simulink model "RCAMSimulation"  (R2025a)
settings: Solver=VariableStepAuto  StartTime=0.0  StopTime=60  RelTol=1e-3
values from neighbouring files (symbols this model uses):
  dt = 1/50    (= 0.02)    [InitializeConstants.m]    (also in joystickdemo.m)
  h0 = 500    [InitializeConstants.m]
  lat0 = deg2rad(21.3245)    [InitializeConstants.m]
  lon0 = deg2rad(-157.9251)    [InitializeConstants.m]
  u1max = 25*pi/180    (= 0.436332312999)    [InitializeConstants.m]    (also in RCAM_model.m)
  u1min = -25*pi/180    (= -0.436332312999)    [InitializeConstants.m]    (also in RCAM_model.m)
  x0 = [85 ... (first row only)    [InitializeConstants.m]
undefined symbols (not defined in the file or in its folder): RCAM_model
libraries: aerolibfltsims x2, aerolibanimutils x1
settings Model: Creator=pjpra  LastModifiedBy=pjpra

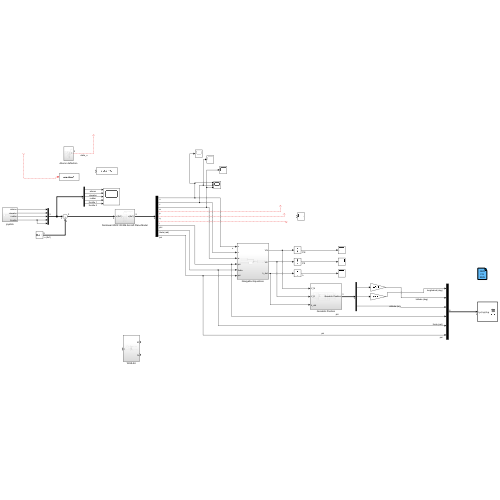
[thumbnail: Simulink's stored preview of the top-level diagram]
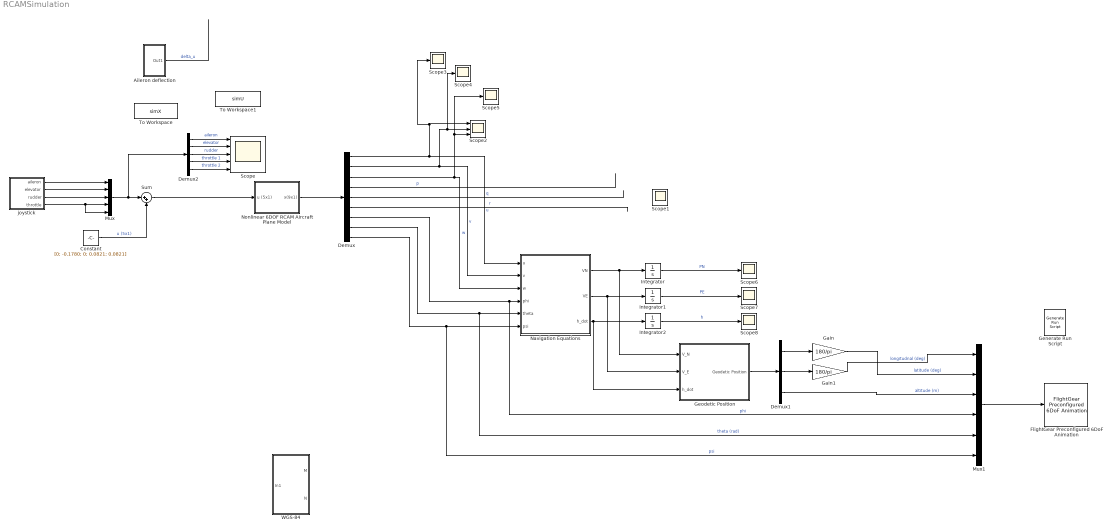
== system RCAMSimulation ==
  Aileron deflection : Subsystem
  Constant : Constant  Value=[0; -0.1780; 0; 0.0821; 0.0821]
  Demux : Demux  Outputs=9
  Demux1 : Demux  Outputs=3
  Demux2 : Demux  Outputs=5
  FlightGear Preconfigured 6DoF Animation : aerolibfltsims/FlightGear Preconfigured 6DoF Animation  xFlightGearVersion=v2019.1  DestinationIpAddress=127.0.0.1  DestinationPort=5502  SampleTime=1/30  packetVersion=24
  Gain : Gain  Gain=180/pi
  Gain1 : Gain  Gain=180/pi
  Generate Run Script : aerolibfltsims/Generate Run Script  Architecture=Win64  dataFlow=Send  GeometryModelName=c172p  AirportId=KSFO  RunwayId=10L  InitialAltitude=7224  InitialHeading=113  OffsetDistance=4.72  OffsetAzimuth=0  InstallScenery=off  DisableShaders=on  OriginAddress=127.0.0.1  DestinationPort=5502  OriginPort=5505  LocalAddress=127.0.0.1  OutputFileName=runfg.bat  FlightGearBaseDirectory=C:\Program Files\FlightGear 2019.1.1
  Geodetic Position : Subsystem
  Integrator : Integrator
  Integrator1 : Integrator
  Integrator2 : Integrator
  Mux : Mux  Inputs=5
  Mux1 : Mux  Inputs=6
  Navigation Equations : Subsystem
  Nonlinear 6DOF RCAM Aircraft Plane Model : Subsystem
  Scope : Scope  NumInputPorts=5
      settings: ActiveDisplayYMinimum=-1  ActiveDisplayYMaximum=1  DataLoggingVariableName=ScopeData3
  Scope{1,3..8} (7 alike) : Scope
      Scope3 settings: ActiveDisplayYMinimum=-115.46318833968678  ActiveDisplayYMaximum=190.41451704390158  DataLoggingVariableName=ScopeData2
      Scope4 settings: ActiveDisplayYMinimum=-115.46318833968678  ActiveDisplayYMaximum=190.41451704390158  DataLoggingVariableName=ScopeData4
      Scope5 settings: ActiveDisplayYMinimum=-115.46318833968678  ActiveDisplayYMaximum=190.41451704390158  DataLoggingVariableName=ScopeData5
      Scope6 settings: ActiveDisplayYMinimum=-336.04878377704415  ActiveDisplayYMaximum=625.66382781010861  DataLoggingVariableName=ScopeData6
      Scope7 settings: ActiveDisplayYMinimum=-115.46318833968678  ActiveDisplayYMaximum=190.41451704390158  DataLoggingVariableName=ScopeData7
      Scope8 settings: ActiveDisplayYMinimum=-228.9226672413669  ActiveDisplayYMaximum=328.44496651210937  DataLoggingVariableName=ScopeData8
  Scope2 : Scope  NumInputPorts=3
      settings: ActiveDisplayYMinimum=-115.46318833968678  ActiveDisplayYMaximum=190.41451704390158
  Sum : Sum  Inputs=|++
  To Workspace : ToWorkspace  VariableName=simX  SaveFormat=Timeseries  SampleTime=-1
  To Workspace1 : ToWorkspace  VariableName=simU  SaveFormat=Timeseries  SampleTime=-1
  WGS-84 : Subsystem
  joystick : Subsystem
  wires:
  Constant/1 -> Sum/2  "u (5x1)"
  ? -> To Workspace/1
  Sum/1 -> Nonlinear 6DOF RCAM Aircraft Plane Model/1(u (5x1))
  Aileron deflection/1(Out1) -> ?  "delta_u"
  Nonlinear 6DOF RCAM Aircraft Plane Model/1(x(9x1)) -> Demux/1
  Demux/9 -> Mux1/6, Navigation Equations/6(psi)  "psi"
  Demux/7 -> Mux1/4, Navigation Equations/4(phi)  "phi"
  Demux/3 -> Scope5/1, Scope2/3, Navigation Equations/3(w)  "w"
  Demux/2 -> Scope4/1, Scope2/2, Navigation Equations/2(v)  "v"
  Demux/1 -> Scope3/1, Scope2/1, Navigation Equations/1(u)  "u"
  Navigation Equations/1(VN) -> Integrator/1, Geodetic Position/1(V_N)
  Navigation Equations/2(VE) -> Integrator1/1, Geodetic Position/2(V_E)
  Navigation Equations/3(h_dot) -> Geodetic Position/3(h_dot), Integrator2/1
  Geodetic Position/1(Geodetic Position) -> Demux1/1
  joystick/1(aileron) -> Mux/1
  joystick/2(elevator) -> Mux/2
  joystick/4(throttle) -> Mux/5, Mux/4
  Mux/1 -> Demux2/1, Sum/1
  Demux2/1 -> Scope/1  "aileron"
  Demux2/2 -> Scope/2  "elevator"
  Demux2/3 -> Scope/3  "rudder"
  Demux2/4 -> Scope/4  "throttle 1"
  Demux2/5 -> Scope/5  "throttle 2"
  joystick/3(rudder) -> Mux/3
  Demux1/1 -> Gain/1
  Demux1/2 -> Gain1/1
  Demux/4 -> ?  "p"
  Demux/5 -> ?  "q"
  Demux/6 -> ?  "r"
  Mux1/1 -> FlightGear Preconfigured 6DoF Animation/1
  Gain1/1 -> Mux1/1  "longitudnal (deg)"
  Gain/1 -> Mux1/2  "latitude (deg)"
  Demux1/3 -> Mux1/3  "altitude (m)"
  Demux/8 -> Mux1/5, Navigation Equations/5(theta)  "theta (rad)"
  Integrator2/1 -> Scope8/1  "h"
  Integrator1/1 -> Scope7/1  "PE"
  Integrator/1 -> Scope6/1  "PN"

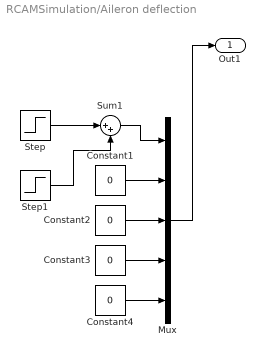
== system RCAMSimulation/Aileron deflection ==
  Constant{1..4} (4 alike) : Constant  Value=0
  Mux : Mux  Inputs=5
  Step : Step  Time=30  After=5*pi/180  SampleTime=0
  Step1 : Step  Time=30+2  After=-5*pi/180  SampleTime=0
  Sum1 : Sum  Inputs=|++
  Out1 : Outport
  wires:
  Constant3/1 -> Mux/4
  Constant1/1 -> Mux/2
  Step/1 -> Sum1/1
  Constant4/1 -> Mux/5
  Constant2/1 -> Mux/3
  Sum1/1 -> Mux/1
  Mux/1 -> Out1/1
  Step1/1 -> Sum1/2

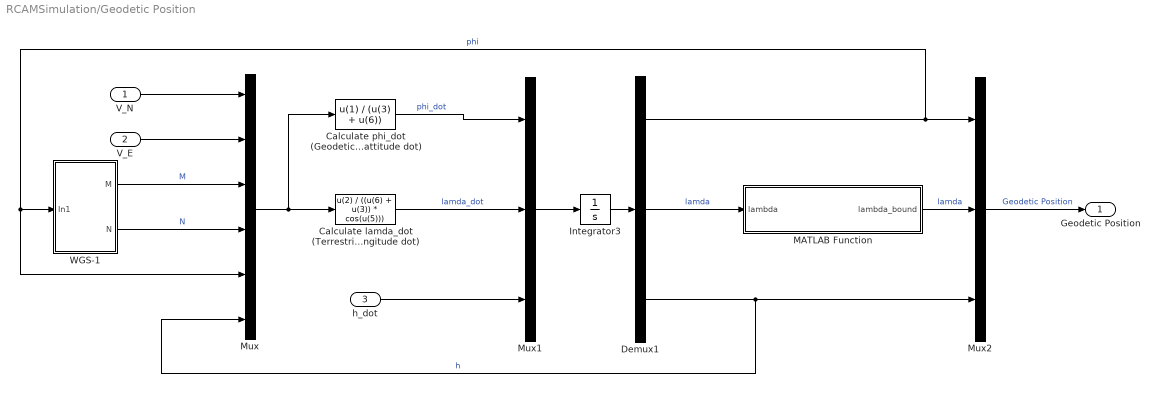
== system RCAMSimulation/Geodetic Position ==
  V_N : Inport
  V_E : Inport  Port=2
  h_dot : Inport  Port=3
  Calculate lamda_dot (Terrestrial Longitude dot) : Fcn  Expr=u(2) / ((u(6) + u(3)) * cos(u(5)))
  Calculate phi_dot (Geodetic Lattitude dot) : Fcn  Expr=u(1) / (u(3) + u(6))
  Demux1 : Demux  Outputs=3
  Integrator3 : Integrator  InitialCondition=[lat0; lon0; h0]
  MATLAB Function : MATLAB Function  TreatAsAtomicUnit=on
  Mux : Mux  Inputs=6
  Mux1 : Mux  Inputs=3
  Mux2 : Mux  Inputs=3
  WGS-1 : Subsystem
  Geodetic Position : Outport
  wires:
  Mux/1 -> Calculate phi_dot (Geodetic Lattitude dot)/1, Calculate lamda_dot (Terrestrial Longitude dot)/1
  Demux1/2 -> MATLAB Function/1(lambda)  "lamda"
  MATLAB Function/1(lambda_bound) -> Mux2/2  "lamda"
  Demux1/1 -> WGS-1/1(In1), Mux/5, Mux2/1  "phi"
  WGS-1/2(N) -> Mux/4  "N"
  Demux1/3 -> Mux/6, Mux2/3  "h"
  Calculate phi_dot (Geodetic Lattitude dot)/1 -> Mux1/1  "phi_dot"
  Mux1/1 -> Integrator3/1
  Calculate lamda_dot (Terrestrial Longitude dot)/1 -> Mux1/2  "lamda_dot"
  Integrator3/1 -> Demux1/1
  WGS-1/1(M) -> Mux/3  "M"
  V_N/1 -> Mux/1
  V_E/1 -> Mux/2
  Mux2/1 -> Geodetic Position/1  "Geodetic Position"
  h_dot/1 -> Mux1/3

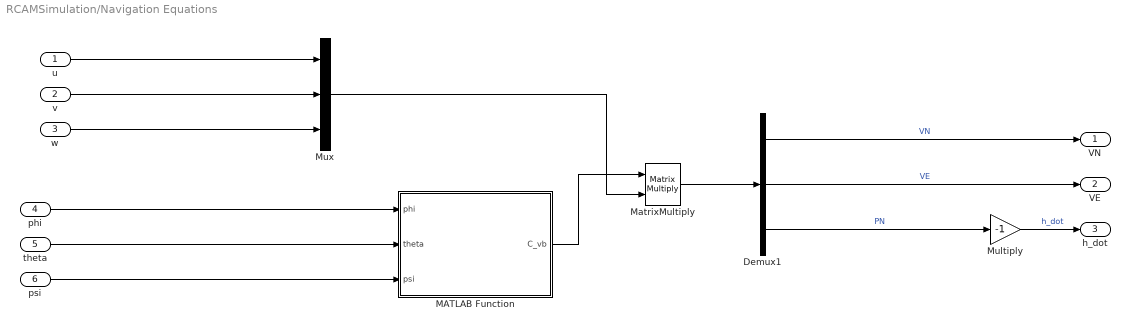
== system RCAMSimulation/Navigation Equations ==
  u : Inport
  v : Inport  Port=2
  w : Inport  Port=3
  phi : Inport  Port=4
  theta : Inport  Port=5
  psi : Inport  Port=6
  Demux1 : Demux  Outputs=3
  MATLAB Function : MATLAB Function  TreatAsAtomicUnit=on
  MatrixMultiply : Product  Multiplication=Matrix(*)
  Multiply : Gain  Gain=-1
  Mux : Mux  Inputs=3
  VN : Outport
  VE : Outport  Port=2
  h_dot : Outport  Port=3
  wires:
  MatrixMultiply/1 -> Demux1/1
  u/1 -> Mux/1
  Demux1/2 -> VE/1  "VE"
  Mux/1 -> MatrixMultiply/2
  MATLAB Function/1(C_vb) -> MatrixMultiply/1
  theta/1 -> MATLAB Function/2(theta)
  Multiply/1 -> h_dot/1  "h_dot"
  psi/1 -> MATLAB Function/3(psi)
  Demux1/3 -> Multiply/1  "PN"
  v/1 -> Mux/2
  phi/1 -> MATLAB Function/1(phi)
  w/1 -> Mux/3
  Demux1/1 -> VN/1  "VN"

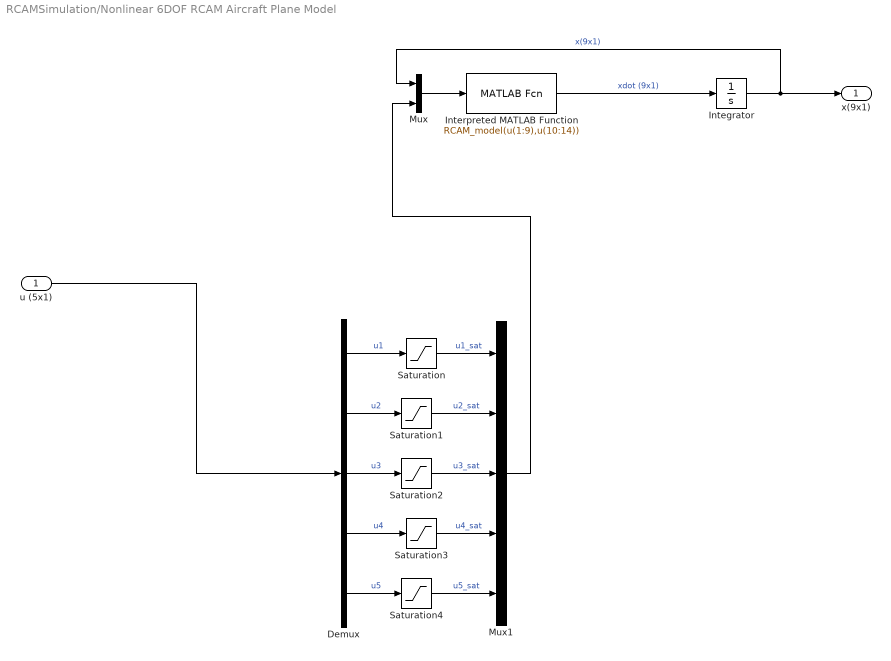
== system RCAMSimulation/Nonlinear 6DOF RCAM Aircraft Plane Model ==
  u (5x1) : Inport
  Demux : Demux  Outputs=5
  Integrator : Integrator  InitialCondition=x0
  Interpreted MATLAB Function : MATLABFcn  MATLABFcn=RCAM_model(u(1:9),u(10:14))
  Mux : Mux  Inputs=2
  Mux1 : Mux  Inputs=5
  Saturation{,1..4} (5 alike) : Saturate  UpperLimit=u1max  LowerLimit=u1min
  x(9x1) : Outport
  wires:
  Integrator/1 -> x(9x1)/1, Mux/1  "x(9x1)"
  Interpreted MATLAB Function/1 -> Integrator/1  "xdot (9x1)"
  Mux/1 -> Interpreted MATLAB Function/1
  Demux/1 -> Saturation/1  "u1"
  Demux/2 -> Saturation1/1  "u2"
  Demux/3 -> Saturation2/1  "u3"
  Demux/4 -> Saturation3/1  "u4"
  Demux/5 -> Saturation4/1  "u5"
  Saturation/1 -> Mux1/1  "u1_sat"
  Saturation1/1 -> Mux1/2  "u2_sat"
  Saturation2/1 -> Mux1/3  "u3_sat"
  Saturation3/1 -> Mux1/4  "u4_sat"
  Saturation4/1 -> Mux1/5  "u5_sat"
  u (5x1)/1 -> Demux/1
  Mux1/1 -> Mux/2

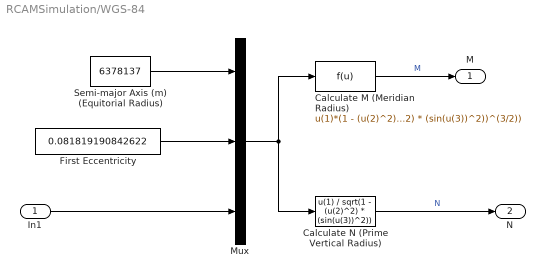
== system RCAMSimulation/WGS-84 ==
  In1 : Inport
  Calculate M (Meridian Radius) : Fcn  Expr=u(1)*(1 - (u(2)^2)) / ((1 - (u(2)^2) * (sin(u(3))^2))^(3/2))
  Calculate N (Prime Vertical Radius) : Fcn  Expr=u(1) / sqrt(1 - (u(2)^2) * (sin(u(3))^2))
  First Eccentricity : Constant  Value=0.081819190842622
  Mux : Mux  Inputs=3
  Semi-major Axis (m) (Equitorial Radius) : Constant  Value=6378137
  M : Outport
  N : Outport  Port=2
  wires:
  Calculate N (Prime Vertical Radius)/1 -> N/1  "N"
  Semi-major Axis (m) (Equitorial Radius)/1 -> Mux/1
  Mux/1 -> Calculate N (Prime Vertical Radius)/1, Calculate M (Meridian Radius)/1
  First Eccentricity/1 -> Mux/2
  Calculate M (Meridian Radius)/1 -> M/1  "M"
  In1/1 -> Mux/3

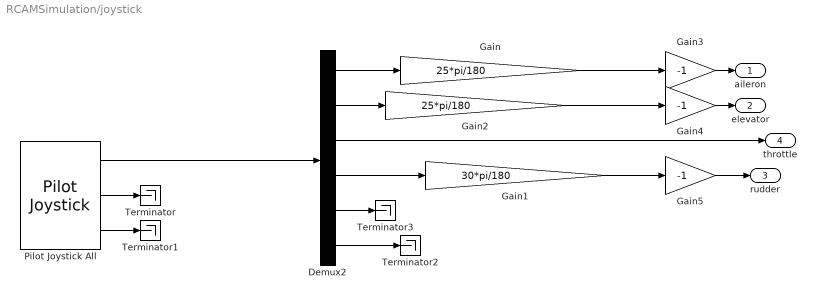
== system RCAMSimulation/joystick ==
  Demux2 : Demux  Outputs=6
  Gain : Gain  Gain=25*pi/180
  Gain1 : Gain  Gain=30*pi/180
  Gain2 : Gain  Gain=25*pi/180
  Gain3 : Gain  Gain=-1
  Gain4 : Gain  Gain=-1
  Gain5 : Gain  Gain=-1
  Pilot Joystick All : aerolibanimutils/Pilot Joystick  JoystickID=Joystick1  OutputConfiguration=AllOutputs  SampleTime=dt
      settings: LibrarySourceBlock=aerolibanimutils/Pilot Joystick All
  Terminator{,1..3} (4 alike) : Terminator
  aileron : Outport
  elevator : Outport  Port=2
  rudder : Outport  Port=3
  throttle : Outport  Port=4
  wires:
  Gain1/1 -> Gain5/1
  Demux2/1 -> Gain/1
  Demux2/4 -> Gain1/1
  Demux2/5 -> Terminator3/1
  Pilot Joystick All/1 -> Demux2/1
  Gain/1 -> Gain3/1
  Demux2/2 -> Gain2/1
  Demux2/6 -> Terminator2/1
  Gain2/1 -> Gain4/1
  Pilot Joystick All/3 -> Terminator1/1
  Pilot Joystick All/2 -> Terminator/1
  Demux2/3 -> throttle/1
  Gain4/1 -> elevator/1
  Gain3/1 -> aileron/1
  Gain5/1 -> rudder/1

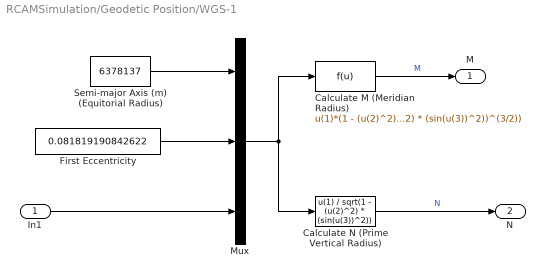
== system RCAMSimulation/Geodetic Position/WGS-1 ==
  In1 : Inport
  Calculate M (Meridian Radius) : Fcn  Expr=u(1)*(1 - (u(2)^2)) / ((1 - (u(2)^2) * (sin(u(3))^2))^(3/2))
  Calculate N (Prime Vertical Radius) : Fcn  Expr=u(1) / sqrt(1 - (u(2)^2) * (sin(u(3))^2))
  First Eccentricity : Constant  Value=0.081819190842622
  Mux : Mux  Inputs=3
  Semi-major Axis (m) (Equitorial Radius) : Constant  Value=6378137
  M : Outport
  N : Outport  Port=2
  wires:
  In1/1 -> Mux/3
  Calculate M (Meridian Radius)/1 -> M/1  "M"
  First Eccentricity/1 -> Mux/2
  Mux/1 -> Calculate M (Meridian Radius)/1, Calculate N (Prime Vertical Radius)/1
  Semi-major Axis (m) (Equitorial Radius)/1 -> Mux/1
  Calculate N (Prime Vertical Radius)/1 -> N/1  "N"

== matlab function RCAMSimulation/Navigation Equations/MATLAB Function ==
  data: phi input; C_vb output; theta input; psi input
function C_vb = calc_C_vb(phi, theta, psi)
% CALC_C_VB  Vehicle-to-Body (NED→Body) Direction Cosine Matrix
%
%   phi   = roll  (rad)
%   theta = pitch (rad)
%   psi   = yaw   (rad)
%
%   The matrix C_vb maps earth-frame (NED) velocity vector [V_N; V_E; V_D]
%   to body-frame velocity vector [u; v; w].
%
%   Relationship:
%       C_vb = (C_bv)';   % transpose of body→vehicle matrix
%
%   Usage:
%       [u; v; w] = C_vb * [V_N; V_E; V_D]
%
%   To go body → vehicle instead, use calc_C_bv(phi,theta,psi).

%#codegen
C_vb = zeros(3,3);

c_phi   = cos(phi);
s_phi   = sin(phi);
c_theta = cos(theta);
s_theta = sin(theta);
c_psi   = cos(psi);
s_psi   = sin(psi);

% Vehicle → Body (transpose of Body → Vehicle)
C_vb(1,1) =  c_theta * c_psi;
C_vb(1,2) =  s_phi * s_theta * c_psi - c_phi * s_psi;
C_vb(1,3) =  c_phi * s_theta * c_psi + s_phi * s_psi;

C_vb(2,1) =  c_theta * s_psi;
C_vb(2,2) =  s_phi * s_theta * s_psi + c_phi * c_psi;
C_vb(2,3) =  c_phi * s_theta * s_psi - s_phi * c_psi;

C_vb(3,1) = -s_theta;
C_vb(3,2) =  s_phi * c_theta;
C_vb(3,3) =  c_phi * c_theta;

end

== matlab function RCAMSimulation/Geodetic Position/MATLAB Function ==
  data: lambda input; lambda_bound output
function lambda_bound = LongitudeBound(lambda)
% Keeps longitude within [-pi, pi]
lambda_bound = wrapToPi(lambda);
end
